simulink model "P3_controlo_atitude"  (R2019a)
settings: Solver=VariableStepAuto  StartTime=0.0  StopTime=T_final  RelTol=1e-3
values from neighbouring files (symbols this model uses):
  A_AA = [ybb  yp+w0/u0 yr-1 g*ctt0/u0 ... (first row only)    [P1.m]    (also in P2.m; P3.m; P3_F.m; P3_serv.m)
  B = [0    ydr ... (first row only)    [P1.m]    (also in P2.m; P3.m; P3_F.m; P3_serv.m)
  bb_ref = 5    [P3.m]    (also in P3_F.m = 0.8; P3_serv.m = 0.8; P3_test.m = 3; P4_F.m = 0.8)
  bb_stept = 10    [P3.m]    (also in P3_F.m; P3_serv.m; P3_test.m; P4_F.m)
  C = eye(4)    [P2.m]    (also in P3.m; P3_F.m; P3_serv.m; P3_test.m)
  D = zeros(4,2)    [P2.m]    (also in P3.m; P3_F.m; P3_serv.m; P3_test.m)
  deg = pi/180    (= 0.0174532925199)    [P1.m]    (also in P2.m; P3.m; P3_F.m; P3_serv.m)
  K_bbphi = [K_lqr(:,1) K_lqr(:,4)]    [P3.m]    (also in P3_serv.m)
  K_int = K_lqr(:,5:6)    [P3.m]    (also in P3_serv.m)
  K_pr = K_lqr(:,2:3)    [P3.m]    (also in P3_serv.m)
  phi_ref = 10    [P3.m]    (also in P3_F.m = 15; P3_serv.m = 8; P3_test.m = 8; P4_F.m = 22)
  phi_stept = 30    [P3.m]    (also in P3_F.m = 50; P3_serv.m = 50; P3_test.m = 50; P4_F.m = 50)
settings Model: Creator=User  LastModifiedBy=tomas
settings DebuggingCC: SFMachineParentedDataDiag=error

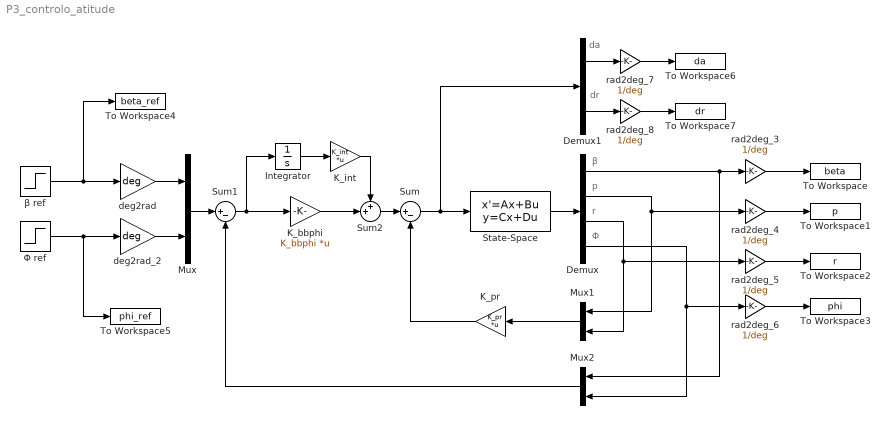
== system P3_controlo_atitude ==
  note: β
  note: p
  note: r
  note: Φ
  note: da
  note: dr
  Demux : Demux
  Demux1 : Demux  Outputs=2
  Integrator : Integrator
  K_bbphi : Gain  Gain=K_bbphi  Multiplication=Matrix(K*u) (u vector)
  K_int : Gain  Gain=K_int  Multiplication=Matrix(K*u) (u vector)
  K_pr : Gain  Gain=K_pr  Multiplication=Matrix(K*u) (u vector)
  Mux : Mux  Inputs=2
  Mux1 : Mux  Inputs=2
  Mux2 : Mux  Inputs=2
  State-Space : StateSpace  A=A_AA  B=B  C=C  D=D  InitialCondition=0
  Sum : Sum  Inputs=|+-
  Sum1 : Sum  Inputs=|+-
  Sum2 : Sum  Inputs=++|
  To Workspace : ToWorkspace  VariableName=beta  SaveFormat=Timeseries  SampleTime=-1
  To Workspace1 : ToWorkspace  VariableName=p  SaveFormat=Timeseries  SampleTime=-1
  To Workspace2 : ToWorkspace  VariableName=r  SaveFormat=Timeseries  SampleTime=-1
  To Workspace3 : ToWorkspace  VariableName=phi  SaveFormat=Timeseries  SampleTime=-1
  To Workspace4 : ToWorkspace  VariableName=beta_ref  SaveFormat=Timeseries  SampleTime=-1
  To Workspace5 : ToWorkspace  VariableName=phi_ref  SaveFormat=Timeseries  SampleTime=-1
  To Workspace6 : ToWorkspace  VariableName=da  SaveFormat=Timeseries  SampleTime=-1
  To Workspace7 : ToWorkspace  VariableName=dr  SaveFormat=Timeseries  SampleTime=-1
  deg2rad : Gain  Gain=deg
  deg2rad_2 : Gain  Gain=deg
  rad2deg_{3..8} (6 alike) : Gain  Gain=1/deg
  Φ ref : Step  Time=phi_stept  After=phi_ref  SampleTime=0
  β ref : Step  Time=bb_stept  After=bb_ref  SampleTime=0
  wires:
  β ref/1 -> To Workspace4/1, deg2rad/1
  Φ ref/1 -> deg2rad_2/1, To Workspace5/1
  deg2rad_2/1 -> Mux/2
  deg2rad/1 -> Mux/1
  State-Space/1 -> Demux/1
  Demux/1 -> Mux2/1, rad2deg_3/1
  Demux/4 -> Mux2/2, rad2deg_6/1
  Demux/2 -> rad2deg_4/1, Mux1/1
  Demux/3 -> rad2deg_5/1, Mux1/2
  Mux1/1 -> K_pr/1
  K_pr/1 -> Sum/2
  Sum/1 -> State-Space/1, Demux1/1
  Mux/1 -> Sum1/1
  Sum1/1 -> Integrator/1, K_bbphi/1
  Mux2/1 -> Sum1/2
  Sum2/1 -> Sum/1
  K_bbphi/1 -> Sum2/2
  Integrator/1 -> K_int/1
  K_int/1 -> Sum2/1
  rad2deg_3/1 -> To Workspace/1
  rad2deg_4/1 -> To Workspace1/1
  rad2deg_5/1 -> To Workspace2/1
  rad2deg_6/1 -> To Workspace3/1
  Demux1/1 -> rad2deg_7/1
  Demux1/2 -> rad2deg_8/1
  rad2deg_7/1 -> To Workspace6/1
  rad2deg_8/1 -> To Workspace7/1
